simulink model "Q3"  (R2018a)
settings: Solver=FixedStepAuto  StartTime=2.0  StopTime=4.5  RelTol=1e-3  EnableMultiTasking=on
libraries: powerlib x40, powerlib_meascontrol x2
settings Model: Creator=ROG  LastModifiedBy=user
settings OptimizationCC: LifeSpan=inf
settings DebuggingCC: SFUnexpectedBacktrackingDiag=warning  SFNoUnconditionalDefaultTransitionDiag=warning  SFExecutionAtInitializationDiag=none
settings CodeAppCC: StateflowObjectComments=on
settings GRTTargetCC: TargetLangStandard=C89/C90 (ANSI)  GeneratePreprocessorConditionals=Disable all
settings ConfigComp: CovMetricSettings=dw  CovHtmlReporting=on  CovSaveCumulativeToWorkspaceVar=on  CovSaveSingleToWorkspaceVar=on  CovExternalEMLEnable=off
settings SimscapeCC: SimscapeNormalizeSystem=off

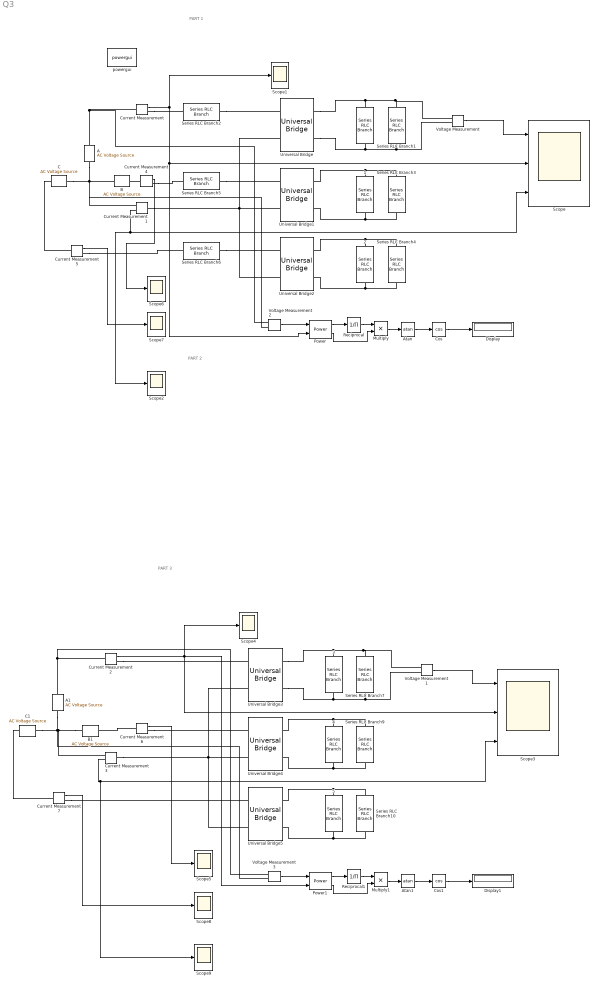
== system Q3 ==
  note: PART 1
  note: PART 2
  note: PART 3
   {,1..5} (6 alike) : powerlib/Elements/Series RLC Branch  LConnTagsString=__new0  RConnTagsString=__new0  BranchType=R  Resistance=200  Inductance=1e-3  SetiL0=off  InitialCurrent=0  Capacitance=1e-6  Setx0=off  InitialVoltage=0  Measurements=None
  A : powerlib/Electrical Sources/AC Voltage Source  Amplitude=325  Phase=0  Frequency=50  SampleTime=0  Measurements=None  BusType=swing  Pref=10e3  Qref=0  Qmin=-inf  Qmax=+inf
  A1 : powerlib/Electrical Sources/AC Voltage Source  Amplitude=325  Phase=0  Frequency=50  SampleTime=0  Measurements=None  BusType=swing  Pref=10e3  Qref=0  Qmin=-inf  Qmax=+inf
  Atan : Trigonometry  Operator=atan
  Atan1 : Trigonometry  Operator=atan
  B : powerlib/Electrical Sources/AC Voltage Source  Amplitude=325  Phase=120  Frequency=50  SampleTime=0  Measurements=None  BusType=swing  Pref=10e3  Qref=0  Qmin=-inf  Qmax=+inf
  B1 : powerlib/Electrical Sources/AC Voltage Source  Amplitude=325  Phase=120  Frequency=50  SampleTime=0  Measurements=None  BusType=swing  Pref=10e3  Qref=0  Qmin=-inf  Qmax=+inf
  C : powerlib/Electrical Sources/AC Voltage Source  Amplitude=325  Phase=240  Frequency=50  SampleTime=0  Measurements=None  BusType=swing  Pref=10e3  Qref=0  Qmin=-inf  Qmax=+inf
  C1 : powerlib/Electrical Sources/AC Voltage Source  Amplitude=325  Phase=240  Frequency=50  SampleTime=0  Measurements=None  BusType=swing  Pref=10e3  Qref=0  Qmin=-inf  Qmax=+inf
  Cos : Trigonometry  Operator=cos
  Cos1 : Trigonometry  Operator=cos
  Current Measurement{,1,4..5} (4 alike) : powerlib/Measurements/Current Measurement  PhasorSimulation=off  OutputType=Complex  PSBequivalent=0
  Current Measurement{2..3,6..7} (4 alike) : powerlib/Measurements/Current Measurement  PhasorSimulation=off  OutputType=Magnitude  PSBequivalent=0
  Display : Display
  Display1 : Display
  Multiply : Product
  Multiply1 : Product
  Power : powerlib_meascontrol/Measurements/Power  Freq=50  Vinit=[1, 0]  Iinit=[1, 0]  Ts=0
      settings: SourceProductName=Simscape Power Systems
  Power1 : powerlib_meascontrol/Measurements/Power  Freq=50  Vinit=[1, 0]  Iinit=[1, 0]  Ts=0
      settings: SourceProductName=Simscape Power Systems
  Reciprocal : Product  Inputs=/
  Reciprocal1 : Product  Inputs=/
  Scope : Scope  NumInputPorts=3
  Scope{1..2,4..9} (8 alike) : Scope
  Scope3 : Scope  NumInputPorts=3
  Series RLC Branch{1,3..4,7,9..10} (6 alike) : powerlib/Elements/Series RLC Branch  LConnTagsString=__new0  RConnTagsString=__new0  BranchType=C  Resistance=1  Inductance=1e-3  SetiL0=off  InitialCurrent=0  Capacitance=470e-6  Setx0=off  InitialVoltage=0  Measurements=None
  Series RLC Branch2 : powerlib/Elements/Series RLC Branch  LConnTagsString=__new0  RConnTagsString=__new0  BranchType=L  Resistance=1  Inductance=600e-6  SetiL0=off  InitialCurrent=0  Capacitance=1e-6  Setx0=off  InitialVoltage=0  Measurements=None
  Series RLC Branch5 : powerlib/Elements/Series RLC Branch  LConnTagsString=__new0  RConnTagsString=__new0  BranchType=L  Resistance=1  Inductance=600e-6  SetiL0=off  InitialCurrent=0  Capacitance=1e-6  Setx0=off  InitialVoltage=0  Measurements=None
  Series RLC Branch6 : powerlib/Elements/Series RLC Branch  LConnTagsString=__new0  RConnTagsString=__new0  BranchType=L  Resistance=1  Inductance=600e-6  SetiL0=off  InitialCurrent=0  Capacitance=1e-6  Setx0=off  InitialVoltage=0  Measurements=None
  Universal Bridge{,1..5} (6 alike) : powerlib/Power Electronics/Universal Bridge  Arms=2  SnubberResistance=1e5  SnubberCapacitance=inf  Device=Diodes  Ron=1e-3  Lon=0  ForwardVoltages="[  0  0  ]"  ForwardVoltage=0  GTOparameters=[ 10e-6 , 20e-6 ]  IGBTparameters=[ 1e-6 , 2e-6 ]  Measurements=None  Measurements_2=None  converterType=Rectifier
  Voltage Measurement{,1..3} (4 alike) : powerlib/Measurements/Voltage Measurement  PhasorSimulation=off  OutputType=Complex  PSBequivalent=0
  powergui : powerlib/powergui  Priority=1  SimulationMode=Discrete  SampleTime=1e-6  frequency=60  Iterations=50  frequencyindice=50  Pbase=100e6  ErrMax=1e-4  UnitsV=kV  UnitsW=MW  buscounter=0  FunctionMessages=off  echomessages=off  EnableUseOfTLC=off  CurrentSourceSwitches=off  DisableSnubberDevices=off  DisableRonSwitches=off  DisableVfSwitches=off  DisplayEquations=off  SolverType=Tustin/Backward Euler (TBE)  Interpol=off  ExternalGateDelay=off  methode=off  Ts=100  x0status=blocks  SPID=off  SwTol=0  HookPort=off  RestoreLinks=warning  ResistiveCurrentMeasurement=off  Frange=[0:2:500]  Ylog=off  Xlog=on  ShowGrid=off  save=off  variable=ZData  structure=InputCurrent  ZoomFFT=off  StartTime=2.3  cycles=100  DisplayStyle=2  fundamental=50  FreqAxis=off  MaxFrequency=1000  frequencyindicesteady=1  RmsSteady=1  display=off
  wires:
  Voltage Measurement/1 -> Scope/1
  Current Measurement/1 -> Power/2, Scope/2, Scope1/1
  Current Measurement1/1 -> Scope/3, Scope2/1
  Current Measurement3/1 -> Scope9/1, Scope3/3
  Voltage Measurement1/1 -> Scope3/1
  Current Measurement2/1 -> Power1/2, Scope4/1, Scope3/2
  Current Measurement4/1 -> Scope6/1
  Current Measurement5/1 -> Scope7/1
  Current Measurement6/1 -> Scope5/1
  Current Measurement7/1 -> Scope8/1
  Voltage Measurement2/1 -> Power/1
  Power/2 -> Multiply/2
  Power/1 -> Reciprocal/1
  Reciprocal/1 -> Multiply/1
  Multiply/1 -> Atan/1
  Atan/1 -> Cos/1
  Cos/1 -> Display/1
  Cos1/1 -> Display1/1
  Voltage Measurement3/1 -> Power1/1
  Multiply1/1 -> Atan1/1
  Reciprocal1/1 -> Multiply1/1
  Power1/1 -> Reciprocal1/1
  Atan1/1 -> Cos1/1
  Power1/2 -> Multiply1/2
  connections:
  C/LConn1 -- Voltage Measurement2/LConn2 -- A/LConn1 -- Current Measurement1/RConn1 -- B/LConn1
  Series RLC Branch2/RConn1 -- Universal Bridge/LConn1
  Series RLC Branch5/RConn1 -- Universal Bridge1/LConn1
  Series RLC Branch6/RConn1 -- Universal Bridge2/LConn1
  Universal Bridge/RConn1 -- " "/LConn1 -- Voltage Measurement/LConn1 -- Series RLC Branch1/LConn1
  Universal Bridge/RConn2 -- Voltage Measurement/LConn2 -- Series RLC Branch1/RConn1 -- " "/RConn1
  " 1"/LConn1 -- Series RLC Branch3/LConn1 -- Universal Bridge1/RConn1
  " 1"/RConn1 -- Universal Bridge1/RConn2 -- Series RLC Branch3/RConn1
  " 2"/LConn1 -- Universal Bridge2/RConn1 -- Series RLC Branch4/LConn1
  " 2"/RConn1 -- Universal Bridge2/RConn2 -- Series RLC Branch4/RConn1
  Current Measurement5/LConn1 -- C/RConn1
  Current Measurement/RConn1 -- Series RLC Branch2/LConn1
  Current Measurement/LConn1 -- Voltage Measurement2/LConn1 -- A/RConn1
  Universal Bridge/LConn2 -- Current Measurement1/LConn1 -- Universal Bridge2/LConn2 -- Universal Bridge1/LConn2
  " 3"/RConn1 -- Universal Bridge3/RConn2 -- Voltage Measurement1/LConn2 -- Series RLC Branch7/RConn1
  Series RLC Branch10/RConn1 -- " 5"/RConn1 -- Universal Bridge5/RConn2
  B1/LConn1 -- Current Measurement3/RConn1 -- Voltage Measurement3/LConn2 -- C1/LConn1 -- A1/LConn1
  Series RLC Branch10/LConn1 -- " 5"/LConn1 -- Universal Bridge5/RConn1
  Series RLC Branch7/LConn1 -- Universal Bridge3/RConn1 -- " 3"/LConn1 -- Voltage Measurement1/LConn1
  Universal Bridge4/LConn2 -- Universal Bridge3/LConn2 -- Current Measurement3/LConn1 -- Universal Bridge5/LConn2
  Universal Bridge4/RConn1 -- " 4"/LConn1 -- Series RLC Branch9/LConn1
  Series RLC Branch9/RConn1 -- " 4"/RConn1 -- Universal Bridge4/RConn2
  Current Measurement2/RConn1 -- Universal Bridge3/LConn1
  Current Measurement2/LConn1 -- Voltage Measurement3/LConn1 -- A1/RConn1
  Current Measurement4/LConn1 -- B/RConn1
  Current Measurement4/RConn1 -- Series RLC Branch5/LConn1
  Current Measurement5/RConn1 -- Series RLC Branch6/LConn1
  Current Measurement6/LConn1 -- B1/RConn1
  Current Measurement6/RConn1 -- Universal Bridge4/LConn1
  Current Measurement7/RConn1 -- Universal Bridge5/LConn1
  C1/RConn1 -- Current Measurement7/LConn1
